simulink model "xpcosc"  (Simulink 7.7)
settings: Solver=ode4  StartTime=0.0  StopTime=0.2  FixedStep=0.001  RelTol=1e-3
undefined symbols (not defined in the file): madnipcim
libraries: xpcnilib x1, xpclib x1
settings Model: Creator=mvetsch  LastModifiedBy=newton  BufferReuse=off
settings DataIOCC: LimitDataPoints=off  SaveState=on  SignalLoggingName=logsOut
settings OptimizationCC: BlockReduction=off  BooleanDataType=off  OptimizeBlockIOStorage=off  BufferReuse=off  ExpressionFolding=off  LocalBlockOutputs=off  InitFltsAndDblsToZero=on
settings DebuggingCC: SaveWithParameterizedLinksMsg=none  CheckExecutionContextPreStartOutputMsg=on  CheckExecutionContextRuntimeOutputMsg=on  SignalResolutionControl=TryResolveAllWithWarning  SolverPrmCheckMsg=none  MultiTaskDSMMsg=warning  MultiTaskCondExecSysMsg=none  StrictBusMsg=None
settings HardwareCC: ProdIntDivRoundTo=Zero  ProdEndianess=LittleEndian  ProdHWDeviceType=Generic->32-bit x86 compatible
settings RTWCC: SystemTargetFile=xpctarget.tlc  TemplateMakefile=xpc_default_tmf  Description=xPC Target  ProcessScript=xpctarget_make_rtw_hook  IncludeERTFirstTime=on  RTWCompilerOptimization=On
settings xpcTargetCC: TargetFcnLib=ansi_tfl_tmw.mat  TargetFunctionLibrary=XPC_BLAS  FunctionExecutionProfile=off  CodeExecutionProfiling=off  ERTCodeCoverageTool=None  ParMdlRefBuildCompliant=on  CombineSignalStateStructs=off  PortableWordSizes=off  xPCTaskExecutionProfile=off  xPCRL32EventNumber=5000  xPCLoadParamSetFile=off  xPCConcurrentTasks=off  xPCEnableSFAnimation=off

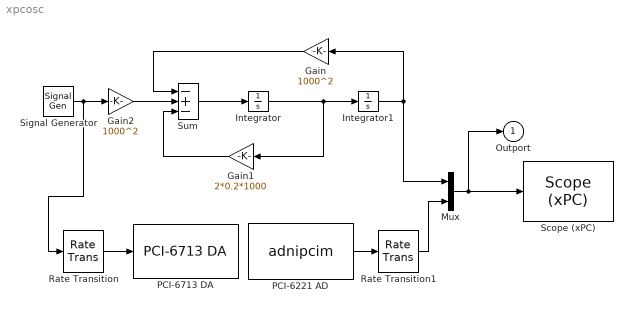
== system xpcosc ==
  Gain : Gain  Gain=1000^2  SaturateOnIntegerOverflow=on  OutDataTypeStr=Inherit: Same as input  ParamDataTypeStr=Inherit: Same as input
  Gain1 : Gain  Gain=2*0.2*1000  SaturateOnIntegerOverflow=on  OutDataTypeStr=Inherit: Same as input  ParamDataTypeStr=Inherit: Same as input
  Gain2 : Gain  Gain=1000^2  SaturateOnIntegerOverflow=on  OutDataTypeStr=Inherit: Same as input  ParamDataTypeStr=Inherit: Same as input
  Integrator : Integrator
  Integrator1 : Integrator
  Mux : Mux  Inputs=2
  PCI-6221 AD : S-Function  AncestorBlock=xpcnilib/A//D/M Series/PCI-6221 AD  InitFcn=madnipcim(1);  FunctionName=adnipcim  Parameters="channel, range, coupling, scantime, sampletime, slot,  boardType"  SFunctionModules=xpcionim  EnableBusSupport=off  mask(adnipci6221){channel=[1], range=[10], coupling=[0], scantime=5e-6, sampletime=0.001, slot=-1}
      mask prompts: channel "Channel vector (1-16):"; range "Range vector (in the set [10, 5, 1, 0.2]):"; coupling "Input coupling vector (0: RSE, 1: NRSE, 2: DIFF):"; scantime "Scan Interval:"; sampletime "Sample time:"; slot "PCI slot (-1: autosearch):"
      mask help:
      | PCI-6221
      | National Instruments
      | Analog Input
      mask init:
      | boardType=20;
      | [maskdisplay, range, coupling, scantime] = madnipcim(2,channel, range, coupling, scantime, boardType);
      | set_param( gcb, 'MaskDisplay', maskdisplay );
      mask Help: helpview(fullfile(docroot, 'mapfiles', 'xpc.map'), 'NationalInstruments_PCI-6221_AD')
      mask Display: disp('PCI-6220\nNational Instr.\nAnalog Input'); port_label('output', 1, '1');
  PCI-6713 DA : xpcnilib/D//A/PCI-6713 DA  channel=[1]  reset=[0]  initval=[0]  sampletime=0.001  pcislot=-1
  Rate Transition : RateTransition
  Rate Transition1 : RateTransition
  "Scope (xPC) " : xpclib/Misc./Scope (xPC)   SystemSampleTime=-1  scopeno=1  scopetype=Target  autostart=on  viewmode=Graphical redraw  formatstr='%15.6f'  grid=on  ylimits=[0,0]  nosamples=250  noprepostsamples=0  interleave=1  triggermode=FreeRun  triggersignal=1  triggerlevel=0.0  triggerslope=Either  triggerscope=1  triggersample=0  filename=data.dat  mode=Lazy  writesize=512  autorestart=off  dynamicfilemode=off  maxwritefilesize=512*1024^2
  Signal Generator : SignalGenerator  WaveForm=square  Amplitude=4  Frequency=20
  Sum : Sum  Inputs=-+-  SaturateOnIntegerOverflow=on  InputSameDT=on  OutDataTypeStr=Inherit: Same as first input
  Outport : Outport  InitialOutput=0
  wires:
  Gain2/1 -> Sum/2
  Gain/1 -> Sum/1
  Sum/1 -> Integrator/1
  Integrator/1 -> Integrator1/1, Gain1/1
  Integrator1/1 -> Gain/1, Mux/1
  Gain1/1 -> Sum/3
  Signal Generator/1 -> Gain2/1, Rate Transition/1
  Mux/1 -> Outport/1, "Scope (xPC) "/1
  Rate Transition/1 -> PCI-6713 DA/1
  PCI-6221 AD/1 -> Rate Transition1/1
  Rate Transition1/1 -> Mux/2
